simulink model "tire_model_drive_force"  (R2016a)
settings: Solver=VariableStepAuto  StartTime=0.0  StopTime=10.0  RelTol=1e-3
values from neighbouring files (symbols this model uses):
  C_alpha = 120000    [dynamics.m]    (also in setup.m; tire_test.m = 197)
  mu = 0.37    [dynamics.m]    (also in setup.m = 0.5; tire_test.m = 1.31)
settings Model: Creator=Cyrus  LastModifiedBy=Cyrus

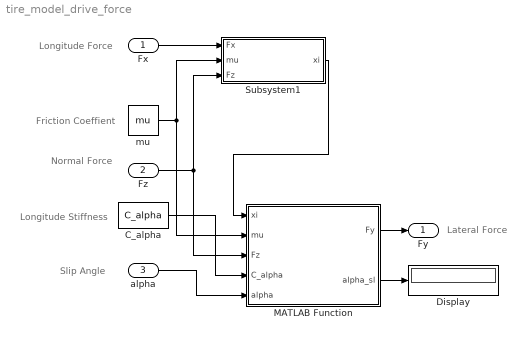
== system tire_model_drive_force ==
  note: Lateral Force
  note: Slip Angle
  note: Longitude Stiffness
  note: Normal Force
  note: Friction Coeffient
  note: Longitude Force
  Fx : Inport
  Fz : Inport  Port=2
  alpha : Inport  Port=3
  C_alpha : Constant  Value=C_alpha
  Display : Display
  MATLAB Function : MATLAB Function  TreatAsAtomicUnit=on
  Subsystem1 : Subsystem
  mu : Constant  Value=mu
  Fy : Outport
  wires:
  Subsystem1/1(xi) -> MATLAB Function/1(xi)
  mu/1 -> Subsystem1/2(mu), MATLAB Function/2(mu)
  Fz/1 -> Subsystem1/3(Fz), MATLAB Function/3(Fz)
  C_alpha/1 -> MATLAB Function/4(C_alpha)
  alpha/1 -> MATLAB Function/5(alpha)
  MATLAB Function/1(Fy) -> Fy/1
  MATLAB Function/2(alpha_sl) -> Display/1
  Fx/1 -> Subsystem1/1(Fx)

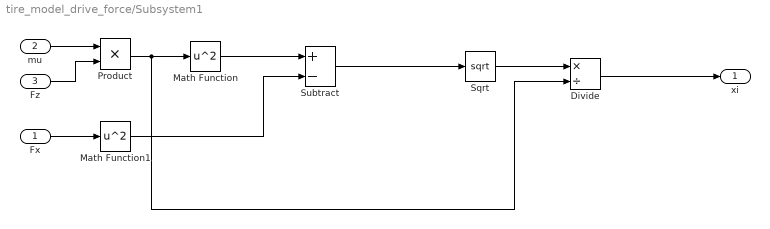
== system tire_model_drive_force/Subsystem1 ==
  Fx : Inport
  mu : Inport  Port=2
  Fz : Inport  Port=3
  Divide : Product  Inputs=*/
  Math Function : Math  Operator=square  SaturateOnIntegerOverflow=on
  Math Function1 : Math  Operator=square  SaturateOnIntegerOverflow=on
  Product : Product
  Sqrt : Sqrt  SaturateOnIntegerOverflow=on
  Subtract : Sum  Inputs=+-
  xi : Outport
  wires:
  mu/1 -> Product/1
  Fz/1 -> Product/2
  Product/1 -> Divide/2, Math Function/1
  Fx/1 -> Math Function1/1
  Math Function/1 -> Subtract/1
  Subtract/1 -> Sqrt/1
  Divide/1 -> xi/1
  Sqrt/1 -> Divide/1
  Math Function1/1 -> Subtract/2

== matlab function tire_model_drive_force/MATLAB Function ==
  data: xi input; mu input; Fz input; C_alpha input; Fy output; alpha input; alpha_sl output
function [Fy, alpha_sl] = fcn(xi, mu, Fz, C_alpha, alpha)
%#codegen
    xi_mu_Fz = xi*mu*Fz;
    alpha_sl = atan(3*xi_mu_Fz/C_alpha);

    tan_alpha = tan(alpha);

    if abs(alpha) <= alpha_sl
        Fy = -C_alpha*tan_alpha+(C_alpha.^2/(3*xi_mu_Fz))*abs(tan_alpha)*tan_alpha-(C_alpha.^3/(27*xi_mu_Fz.^2))*tan_alpha.^3;
    else
        Fy = -xi_mu_Fz*sign(alpha);
    end
end
